simulink model "three_phase_pwm_rectifier_ac_dc_conv_simscape"  (R2019a)
settings: Solver=ode23t  StartTime=0.0  StopTime=1  MaxStep=1e-6  RelTol=1e-6
libraries: powerlib x31, powerlib_meascontrol x1
settings Model: Creator=Görkem  LastModifiedBy=Görkem
settings DataIOCC: ReturnWorkspaceOutputs=off
settings DebuggingCC: ParameterOverflowMsg=none

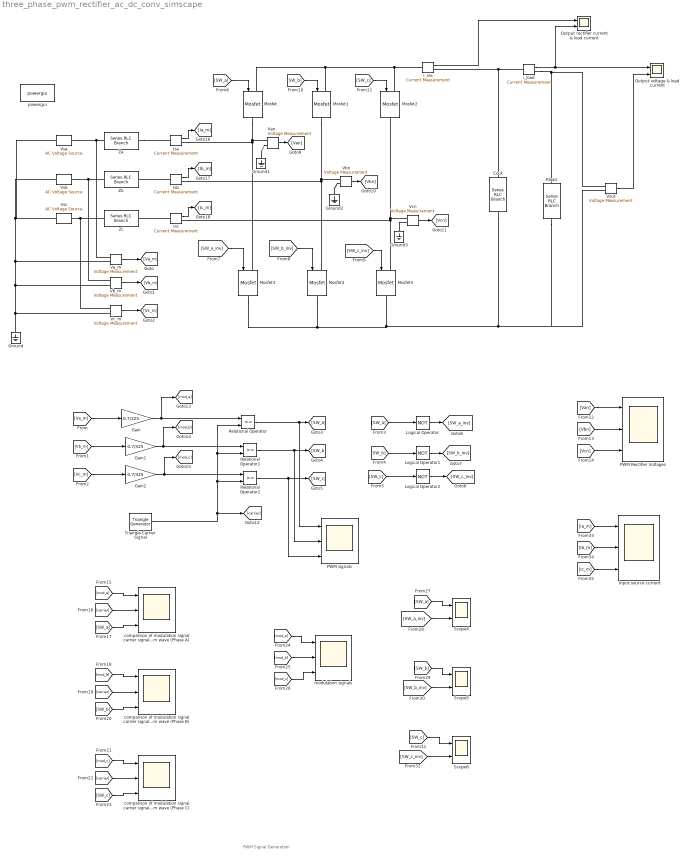
== system three_phase_pwm_rectifier_ac_dc_conv_simscape ==
  note: PWM Signal Generation
  Cout : powerlib/Elements/Series RLC Branch  LConnTagsString=__new0  RConnTagsString=__new0  BranchType=C  Resistance=1  Inductance=1e-3  SetiL0=off  InitialCurrent=0  Capacitance=1000e-6  Setx0=off  InitialVoltage=0  Measurements=None
      settings: SourceProductName=Simscape Electrical
  Gain : Gain  Gain=0.7/325
  Gain1 : Gain  Gain=0.7/325
  Gain2 : Gain  Gain=0.7/325
  Ground{,1..3} (4 alike) : powerlib/Elements/Ground  LConnTagsString=a
      settings: SourceProductName=Simscape Electrical
  I_rec : powerlib/Measurements/Current Measurement  PhasorSimulation=off  OutputType=Complex  PSBequivalent=0
      settings: SourceProductName=Simscape Electrical
  Input source current : Scope  NumInputPorts=3
  Isa : powerlib/Measurements/Current Measurement  PhasorSimulation=off  OutputType=Complex  PSBequivalent=0
      settings: SourceProductName=Simscape Electrical
  Isb : powerlib/Measurements/Current Measurement  PhasorSimulation=off  OutputType=Complex  PSBequivalent=0
      settings: SourceProductName=Simscape Electrical
  Isc : powerlib/Measurements/Current Measurement  PhasorSimulation=off  OutputType=Complex  PSBequivalent=0
      settings: SourceProductName=Simscape Electrical
  Logical Operator : Logic  Operator=NOT  AllPortsSameDT=off  OutDataTypeStr=boolean
  Logical Operator1 : Logic  Operator=NOT  AllPortsSameDT=off  OutDataTypeStr=boolean
  Logical Operator2 : Logic  Operator=NOT  AllPortsSameDT=off  OutDataTypeStr=boolean
  Mosfet{,1..5} (6 alike) : powerlib/Power Electronics/Mosfet  Ron=0.1  Lon=0  Rd=0.01  Vfd=0  IC=0  Rs=1e5  Cs=inf  Measurements=off
      settings: SourceProductName=Simscape Electrical
  Output rectifier current & load current : Scope  NumInputPorts=2
  Output voltage & load current : Scope  NumInputPorts=2
  PWM Rectifier Voltages : Scope  NumInputPorts=3
  PWM signals : Scope  NumInputPorts=3
  Relational Operator : RelationalOperator  OutDataTypeStr=boolean  RndMeth=Simplest
  Relational Operator1 : RelationalOperator  OutDataTypeStr=boolean  RndMeth=Simplest
  Relational Operator2 : RelationalOperator  OutDataTypeStr=boolean  RndMeth=Simplest
  Rload : powerlib/Elements/Series RLC Branch  LConnTagsString=__new0  RConnTagsString=__new0  BranchType=R  Resistance=5  Inductance=1e-3  SetiL0=off  InitialCurrent=0  Capacitance=500e-6  Setx0=off  InitialVoltage=0  Measurements=None
      settings: SourceProductName=Simscape Electrical
  Scope4 : Scope  NumInputPorts=2
  Scope5 : Scope  NumInputPorts=2
  Scope6 : Scope  NumInputPorts=2
  Triangle Carrier Signal : powerlib_meascontrol/Pulse & Signal Generators/Triangle Generator  Freq=10e3  Phase=-90  Ts=0
      settings: SourceProductName=Simscape Electrical
  Va_m : powerlib/Measurements/Voltage Measurement  PhasorSimulation=off  OutputType=Complex  PSBequivalent=0
      settings: SourceProductName=Simscape Electrical
  Van : powerlib/Measurements/Voltage Measurement  PhasorSimulation=off  OutputType=Complex  PSBequivalent=0
      settings: SourceProductName=Simscape Electrical
  Vb_m : powerlib/Measurements/Voltage Measurement  PhasorSimulation=off  OutputType=Complex  PSBequivalent=0
      settings: SourceProductName=Simscape Electrical
  Vbn : powerlib/Measurements/Voltage Measurement  PhasorSimulation=off  OutputType=Complex  PSBequivalent=0
      settings: SourceProductName=Simscape Electrical
  Vc_m : powerlib/Measurements/Voltage Measurement  PhasorSimulation=off  OutputType=Complex  PSBequivalent=0
      settings: SourceProductName=Simscape Electrical
  Vcn : powerlib/Measurements/Voltage Measurement  PhasorSimulation=off  OutputType=Complex  PSBequivalent=0
      settings: SourceProductName=Simscape Electrical
  Vout : powerlib/Measurements/Voltage Measurement  PhasorSimulation=off  OutputType=Complex  PSBequivalent=0
      settings: SourceProductName=Simscape Electrical
  Vsa : powerlib/Electrical Sources/AC Voltage Source  Amplitude=325  Phase=0  Frequency=50  SampleTime=0  Measurements=None  BusType=swing  Pref=10e3  Qref=0  Qmin=-inf  Qmax=+inf
      settings: SourceProductName=Simscape Electrical
  Vsb : powerlib/Electrical Sources/AC Voltage Source  Amplitude=325  Phase=120  Frequency=50  SampleTime=0  Measurements=None  BusType=swing  Pref=10e3  Qref=0  Qmin=-inf  Qmax=+inf
      settings: SourceProductName=Simscape Electrical
  Vsc : powerlib/Electrical Sources/AC Voltage Source  Amplitude=325  Phase=240  Frequency=50  SampleTime=0  Measurements=None  BusType=swing  Pref=10e3  Qref=0  Qmin=-inf  Qmax=+inf
      settings: SourceProductName=Simscape Electrical
  Za : powerlib/Elements/Series RLC Branch  LConnTagsString=__new0  RConnTagsString=__new0  BranchType=RL  Resistance=0.5  Inductance=1e-3  SetiL0=off  InitialCurrent=0  Capacitance=1e-6  Setx0=off  InitialVoltage=0  Measurements=None
      settings: SourceProductName=Simscape Electrical
  Zb : powerlib/Elements/Series RLC Branch  LConnTagsString=__new0  RConnTagsString=__new0  BranchType=RL  Resistance=0.5  Inductance=1e-3  SetiL0=off  InitialCurrent=0  Capacitance=1e-6  Setx0=off  InitialVoltage=0  Measurements=None
      settings: SourceProductName=Simscape Electrical
  Zc : powerlib/Elements/Series RLC Branch  LConnTagsString=__new0  RConnTagsString=__new0  BranchType=RL  Resistance=0.5  Inductance=1e-3  SetiL0=off  InitialCurrent=0  Capacitance=1e-6  Setx0=off  InitialVoltage=0  Measurements=None
      settings: SourceProductName=Simscape Electrical
  comparison of modulation signal carrier signal and pwm wave (Phase A) : Scope  NumInputPorts=3
  comparison of modulation signal carrier signal and pwm wave (Phase B) : Scope  NumInputPorts=3
  comparison of modulation signal carrier signal and pwm wave (Phase C) : Scope  NumInputPorts=3
  i_load : powerlib/Measurements/Current Measurement  PhasorSimulation=off  OutputType=Complex  PSBequivalent=0
      settings: SourceProductName=Simscape Electrical
  modulation signals : Scope  NumInputPorts=3
  powergui : powerlib/powergui  Priority=1  SimulationMode=Continuous  SampleTime=50e-6  frequency=60  Iterations=50  frequencyindice=50  Pbase=100e6  ErrMax=1e-4  UnitsV=kV  UnitsW=MW  buscounter=0  FunctionMessages=off  echomessages=off  EnableUseOfTLC=off  CurrentSourceSwitches=off  DisableSnubberDevices=off  DisableRonSwitches=off  DisableVfSwitches=off  DisplayEquations=off  AutomaticDiscreteSolvers=off  SolverType=Tustin/Backward Euler (TBE)  Interpol=off  ExternalGateDelay=off  methode=off  Ts=100  x0status=blocks  SPID=on  SwTol=0  HookPort=off  NonlinearTolerance=0  nMaxIteration=15  ContinueOnMaxIteration=off  RestoreLinks=warning  ResistiveCurrentMeasurement=off  Frange=[0:2:500]  Ylog=off  Xlog=on  ShowGrid=off  save=off  variable=ZData  structure=0  ZoomFFT=off  StartTime=0.0  cycles=1  DisplayStyle=1  fundamental=60  FreqAxis=off  MaxFrequency=1000  frequencyindicesteady=1  RmsSteady=1  display=off
      settings: SourceProductName=Simscape Electrical
  wires:
  Va_m/1 -> [Va_m]
  Vb_m/1 -> [Vb_m]
  Vc_m/1 -> [Vc_m]
  [Va_m] -> Gain/1
  [Vb_m] -> Gain1/1
  [Vc_m] -> Gain2/1
  Triangle Carrier Signal/1 -> [carrier], Relational Operator2/2, Relational Operator1/2, Relational Operator/2
  Gain1/1 -> [mod_b], Relational Operator1/1
  Gain2/1 -> [mod_c], Relational Operator2/1
  Relational Operator/1 -> PWM signals/1, [SW_a]
  Relational Operator1/1 -> PWM signals/2, [SW_b]
  Relational Operator2/1 -> PWM signals/3, [SW_c]
  [SW_a] -> Logical Operator/1
  [SW_c] -> Logical Operator2/1
  [SW_b] -> Logical Operator1/1
  Logical Operator/1 -> [SW_a_inv]
  Logical Operator1/1 -> [SW_b_inv]
  Logical Operator2/1 -> [SW_c_inv]
  [SW_a] -> Mosfet/1
  [SW_a_inv] -> Mosfet3/1
  [SW_b_inv] -> Mosfet4/1
  [SW_c_inv] -> Mosfet5/1
  Vout/1 -> Output voltage & load current/2
  i_load/1 -> Output rectifier current & load current/2, Output voltage & load current/1
  I_rec/1 -> Output rectifier current & load current/1
  [SW_b] -> Mosfet1/1
  [SW_c] -> Mosfet2/1
  Van/1 -> [Van]
  Vbn/1 -> [Vbn]
  Vcn/1 -> [Vcn]
  [Van] -> PWM Rectifier Voltages/1
  [Vbn] -> PWM Rectifier Voltages/2
  [Vcn] -> PWM Rectifier Voltages/3
  Gain/1 -> Relational Operator/1, [mod_a]
  [mod_a] -> comparison of modulation signal carrier signal and pwm wave (Phase A)/1
  [carrier] -> comparison of modulation signal carrier signal and pwm wave (Phase A)/2
  [SW_a] -> comparison of modulation signal carrier signal and pwm wave (Phase A)/3
  [SW_b] -> comparison of modulation signal carrier signal and pwm wave (Phase B)/3
  [mod_b] -> comparison of modulation signal carrier signal and pwm wave (Phase B)/1
  [carrier] -> comparison of modulation signal carrier signal and pwm wave (Phase B)/2
  [SW_c] -> comparison of modulation signal carrier signal and pwm wave (Phase C)/3
  [mod_c] -> comparison of modulation signal carrier signal and pwm wave (Phase C)/1
  [carrier] -> comparison of modulation signal carrier signal and pwm wave (Phase C)/2
  [mod_b] -> modulation signals/2
  [mod_a] -> modulation signals/1
  [mod_c] -> modulation signals/3
  [SW_a] -> Scope4/1
  [SW_a_inv] -> Scope4/2
  [SW_b] -> Scope5/1
  [SW_b_inv] -> Scope5/2
  [SW_c_inv] -> Scope6/2
  [SW_c] -> Scope6/1
  Isa/1 -> [Ia_m]
  Isb/1 -> [Ib_m]
  Isc/1 -> [Ic_m]
  [Ia_m] -> Input source current/1
  [Ib_m] -> Input source current/2
  [Ic_m] -> Input source current/3
  connections:
  Ground/LConn1 -- Vb_m/LConn2 -- Vsb/LConn1 -- Vsa/LConn1 -- Vsc/LConn1 -- Va_m/LConn2 -- Vc_m/LConn2
  Vsa/RConn1 -- Va_m/LConn1 -- Za/LConn1
  Vsb/RConn1 -- Vb_m/LConn1 -- Zb/LConn1
  Vsc/RConn1 -- Vc_m/LConn1 -- Zc/LConn1
  Mosfet5/LConn1 -- Vcn/LConn1 -- Mosfet2/RConn1 -- Isc/RConn1
  Mosfet1/RConn1 -- Isb/RConn1 -- Mosfet4/LConn1 -- Vbn/LConn1
  Mosfet/RConn1 -- Mosfet3/LConn1 -- Isa/RConn1 -- Van/LConn1
  Mosfet3/RConn1 -- Mosfet4/RConn1 -- Rload/RConn1 -- Vout/LConn2 -- Cout/RConn1 -- Mosfet5/RConn1
  Mosfet/LConn1 -- Mosfet1/LConn1 -- I_rec/LConn1 -- Mosfet2/LConn1
  Cout/LConn1 -- i_load/LConn1 -- I_rec/RConn1
  i_load/RConn1 -- Vout/LConn1 -- Rload/LConn1
  Ground1/LConn1 -- Van/LConn2
  Ground2/LConn1 -- Vbn/LConn2
  Ground3/LConn1 -- Vcn/LConn2
  Za/RConn1 -- Isa/LConn1
  Isb/LConn1 -- Zb/RConn1
  Isc/LConn1 -- Zc/RConn1
